simulink model "practica12"  (R2015a)
settings: Solver=ode45  StartTime=0.0  StopTime=30  RelTol=1e-3
values from neighbouring files (symbols this model uses):
  B = [0;0;0;0;0;(1/m3)]    [practica10cc.m]    (also in practica16.m = [0;1]; practica17.m = [0;1/(m*l*l)]; practica18.m = 1; practica27.m = 1)
  T = 2    [practica27.m]    (also in practica29.m = t(i)-L)
settings Model: Creator=Sala8  LastModifiedBy=Sala8

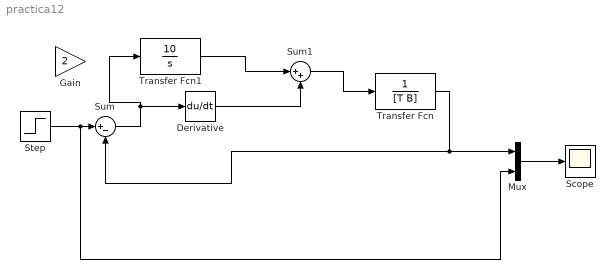
== system practica12 ==
  Derivative : Derivative
  Gain : Gain  Gain=2
  Mux : Mux  Inputs=2
  Scope : Scope
  Step : Step  Time=0  SampleTime=0
  Sum : Sum  Inputs=|+-
  Sum1 : Sum  Inputs=|++
  Transfer Fcn : TransferFcn  Denominator=[T B]
  Transfer Fcn1 : TransferFcn  Numerator=[10]  Denominator=[1 0]
  wires:
  Transfer Fcn/1 -> Sum/2, Mux/1
  Step/1 -> Mux/2, Sum/1
  Mux/1 -> Scope/1
  Sum/1 -> Transfer Fcn1/1, Derivative/1
  Derivative/1 -> Sum1/2
  Transfer Fcn1/1 -> Sum1/1
  Sum1/1 -> Transfer Fcn/1
